simulink model "codd_pfb_fir_4096ch_core"  (R2013b)
settings: Solver=ode45  StartTime=0.0  StopTime=10.0  RelTol=1e-3
undefined symbols (not defined in the file): pfb_coeff_gen_calc
libraries: xbsIndex_r4 x1491, casper_library_misc x112
(part 1 of 18)
settings Model: Creator=ptcs  LastModifiedBy=peix
settings OptimizationCC: ExpressionDepthLimit=2147483647
settings DebuggingCC: StateNameClashWarn=warning

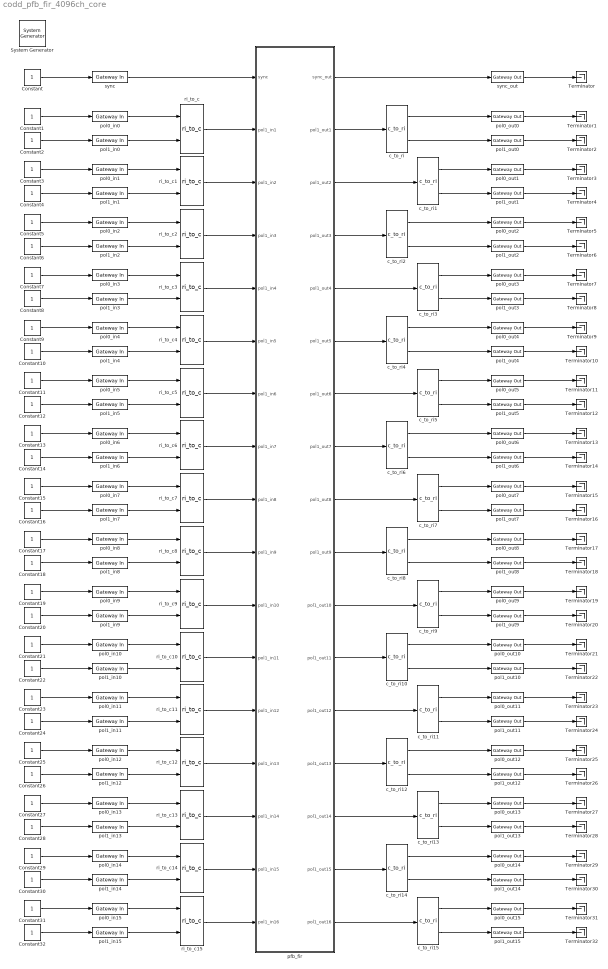
== system codd_pfb_fir_4096ch_core ==
  " System Generator" : xbsIndex_r4/ System Generator  Tag=genX  xilinxfamily=virtex6  part=xc6vsx475t  speed=-1  package=ff1759  synthesis_tool=XST  clock_wrapper=Clock Enables  directory=./codd_pfb_fir_4096ch_core  proj_type=Project Navigator  Synth_file=XST Defaults  Impl_file=ISE Defaults  testbench=off  simulink_period=1  sysclk_period=5.3333  dcm_input_clock_period=100  incr_netlist=off  trim_vbits=Everywhere in SubSystem  dbl_ovrd=According to Block Masks  core_generation=According to Block Masks  run_coregen=off  deprecated_control=off  eval_field=0  block_type=sysgen
  Constant{,1..32} (33 alike) : Constant
  Terminator{,1..32} (33 alike) : Terminator
  c_to_ri{,1..15} (16 alike) : casper_library_misc/c_to_ri  n_bits=18  bin_pt=17
  pfb_fir : Subsystem  Tag=casper:pfb_fir  AncestorBlock=casper_library_pfbs/pfb_fir  mask(pfb_fir){PFBSize=13, TotalTaps=4, WindowType=hamming, n_inputs=4, MakeBiplex=off, BitWidthIn=8, BitWidthOut=18, CoeffBitWidth=18, CoeffDistMem=off, add_latency=1, mult_latency=2, bram_latency=3, fan_latency=2, quantization=Round  (unbiased: Even Values), fwidth=1, mult_spec=2, coeffs_share=on}
      mask prompts: PFBSize "Size of PFB: (2^? pnts)"; TotalTaps "Total Number of Taps:"; WindowType "Windowing Function:"; n_inputs "Number of Simultaneous Inputs: (2^?)"; MakeBiplex "Make Biplex?"; BitWidthIn "Input Bitwidth:"; BitWidthOut "Output Bitwidth:"; CoeffBitWidth "Coefficient Bitwidth:"; CoeffDistMem "Use Distributed Memory for Coeffs"; add_latency "Add Latency"; mult_latency "Mult Latency"; bram_latency "BRAM Latency"; fan_latency "Fanout Latency"; quantization "Quantization Behavior"; fwidth "Bin Width Scaling (normal=1)"; mult_spec "Multiplier specification (0=core, 1=embedded, 2=behavioural) (left=1st tap, or just one value)"; coeffs_share "Share coefficients between polarisations (use less BRAM)?"
      mask init:
      | pfb_fir_init(gcb, ...
      |     'PFBSize', PFBSize, ...
      |     'TotalTaps', TotalTaps, ...
      |     'WindowType', WindowType, ...
      |     'n_inputs', n_inputs, ...
      |     'MakeBiplex', MakeBiplex, ...
      |     'BitWidthIn', BitWidthIn, ...
      |     'BitWidthOut', BitWidthOut, ...
      |     'CoeffBitWidth', CoeffBitWidth, ...
      |     'CoeffDistMem', CoeffDistMem, ...
      |     'add_latency', add_latency, ...
      |     'mult_latency', mult_latency, ...
      |     'bram_latency', bram_latency, ...
      |     'fan_latency', fan_latency, ...
      |     'quantization', quantization, ...
      |     'fwidth', fwidth, ...
      |     'mult_spec', mult_spec, ...
      |     'coeffs_share', coeffs_share);
      settings: AttributesFormatString=|
      | taps=4, add_latency=1
      | max scale 0.596
      mask Help: eval('xlWeb(''http://casper.berkeley.edu/wiki/Pfb_fir'')')
      mask Callback TotalTaps:
      | %num_taps = eval(get_param(gcb, 'TotalTaps'));
      | %old_vec = eval(get_param(gcb, 'mult_spec'));
      | 
      | %vec = 2.*ones(1,num_taps);
      | %old_size = length(old_vec);
      | 
      | %if(old_size <= num_taps),
      | %   new_size = old_size;
      | %else,
      | %    new_size = num_taps;
      | %end
      | 
      | %for n = 1:new_size, vec(n) = old_vec(n); end
      | %set_param(gcb, 'mult_spec', mat2str(vec));
      mask TypeOptions WindowType: bartlett | barthannwin | blackman | blackmanharris | bohamwin | chebwin | flattopwin | gausswin | hamming | hann | kaiser | nuttallwin | parzenwin | rectwin | tukeywin | triang | userwindow
      mask TypeOptions quantization: Truncate | Round  (unbiased: +/- Inf) | Round  (unbiased: Even Values)
      mask Callback fwidth:
      | %num_taps = eval(get_param(gcb, 'TotalTaps'));
      | %old_vec = eval(get_param(gcb, 'mult_spec'));
      | 
      | %vec = 2.*ones(1,num_taps);
      | %old_size = length(old_vec);
      | 
      | %if(old_size <= num_taps),
      | %    new_size = old_size;
      | %else,
      | %    new_size = num_taps;
      | %end
      | 
      | %for n = 1:new_size, vec(n) = old_vec(n); end
      | %set_param(gcb, 'mult_spec', mat2str(vec));
      mask Callback mult_spec:
      | %num_taps = eval(get_param(gcb, 'TotalTaps'));
      | %old_vec = eval(get_param(gcb, 'mult_spec'));
      | 
      | %vec = 2.*ones(1,num_taps);
      | %old_size = length(old_vec);
      | 
      | %if(old_size <= num_taps),
      | %    new_size = old_size;
      | %else,
      | %    new_size = num_taps;
      | %end
      | 
      | %for n = 1:new_size, vec(n) = old_vec(n); end
      | %set_param(gcb, 'mult_spec', mat2str(vec));
  pol0_in{0..15} (16 alike) : xbsIndex_r4/Gateway In  gui_display_data_type=Fixed-point  arith_type="Signed  (2's comp)"  n_bits=8  bin_pt=7  preci_type=Single  exp_width=8  frac_width=24  quantization="Round  (unbiased: +/- Inf)"  overflow=Saturate  period=1  dbl_ovrd=off  timing_constraint=None  locs_specified=off  LOCs={}  UseAsADC=off  ADCChannel='1'  inherit_from_input=off  hdl_port=on  block_type=gatewayin
  pol0_out{0..15} (16 alike) : xbsIndex_r4/Gateway Out  inherit_from_input=off  hdl_port=on  timing_constraint=None  locs_specified=off  LOCs={}  UseAsDAC=off  DACChannel='1'  block_type=gatewayout
  pol1_in{0..15} (16 alike) : xbsIndex_r4/Gateway In  gui_display_data_type=Fixed-point  arith_type="Signed  (2's comp)"  n_bits=8  bin_pt=7  preci_type=Single  exp_width=8  frac_width=24  quantization="Round  (unbiased: +/- Inf)"  overflow=Saturate  period=1  dbl_ovrd=off  timing_constraint=None  locs_specified=off  LOCs={}  UseAsADC=off  ADCChannel='1'  inherit_from_input=off  hdl_port=on  block_type=gatewayin
  pol1_out{0..15} (16 alike) : xbsIndex_r4/Gateway Out  inherit_from_input=off  hdl_port=on  timing_constraint=None  locs_specified=off  LOCs={}  UseAsDAC=off  DACChannel='1'  block_type=gatewayout
  ri_to_c{,1..15} (16 alike) : casper_library_misc/ri_to_c
  sync : xbsIndex_r4/Gateway In  gui_display_data_type=Boolean  arith_type=Boolean  n_bits=16  bin_pt=14  preci_type=Single  exp_width=8  frac_width=24  quantization="Round  (unbiased: +/- Inf)"  overflow=Saturate  period=1  dbl_ovrd=off  timing_constraint=None  locs_specified=off  LOCs={}  UseAsADC=off  ADCChannel='1'  inherit_from_input=off  hdl_port=on  block_type=gatewayin
  sync_out : xbsIndex_r4/Gateway Out  inherit_from_input=off  hdl_port=on  timing_constraint=None  locs_specified=off  LOCs={}  UseAsDAC=off  DACChannel='1'  block_type=gatewayout
  wires:
  pol0_in0/1 -> ri_to_c/1
  pol1_in0/1 -> ri_to_c/2
  ri_to_c/1 -> pfb_fir/2(pol1_in1)
  sync/1 -> pfb_fir/1(sync)
  ri_to_c2/1 -> pfb_fir/4(pol1_in3)
  pol0_in1/1 -> ri_to_c1/1
  pol1_in1/1 -> ri_to_c1/2
  pol0_in2/1 -> ri_to_c2/1
  pol1_in2/1 -> ri_to_c2/2
  ri_to_c1/1 -> pfb_fir/3(pol1_in2)
  ri_to_c3/1 -> pfb_fir/5(pol1_in4)
  pol0_in3/1 -> ri_to_c3/1
  pol1_in3/1 -> ri_to_c3/2
  ri_to_c4/1 -> pfb_fir/6(pol1_in5)
  pol0_in4/1 -> ri_to_c4/1
  pol1_in4/1 -> ri_to_c4/2
  ri_to_c5/1 -> pfb_fir/7(pol1_in6)
  pol0_in5/1 -> ri_to_c5/1
  pol1_in5/1 -> ri_to_c5/2
  ri_to_c6/1 -> pfb_fir/8(pol1_in7)
  pol0_in6/1 -> ri_to_c6/1
  pol1_in6/1 -> ri_to_c6/2
  ri_to_c7/1 -> pfb_fir/9(pol1_in8)
  pol0_in7/1 -> ri_to_c7/1
  pol1_in7/1 -> ri_to_c7/2
  ri_to_c8/1 -> pfb_fir/10(pol1_in9)
  pol0_in8/1 -> ri_to_c8/1
  pol1_in8/1 -> ri_to_c8/2
  ri_to_c9/1 -> pfb_fir/11(pol1_in10)
  pol0_in9/1 -> ri_to_c9/1
  pol1_in9/1 -> ri_to_c9/2
  ri_to_c10/1 -> pfb_fir/12(pol1_in11)
  pol0_in10/1 -> ri_to_c10/1
  pol1_in10/1 -> ri_to_c10/2
  ri_to_c11/1 -> pfb_fir/13(pol1_in12)
  pol0_in11/1 -> ri_to_c11/1
  pol1_in11/1 -> ri_to_c11/2
  ri_to_c12/1 -> pfb_fir/14(pol1_in13)
  pol0_in12/1 -> ri_to_c12/1
  pol1_in12/1 -> ri_to_c12/2
  ri_to_c13/1 -> pfb_fir/15(pol1_in14)
  pol0_in13/1 -> ri_to_c13/1
  pol1_in13/1 -> ri_to_c13/2
  ri_to_c14/1 -> pfb_fir/16(pol1_in15)
  pol0_in14/1 -> ri_to_c14/1
  pol1_in14/1 -> ri_to_c14/2
  ri_to_c15/1 -> pfb_fir/17(pol1_in16)
  pol0_in15/1 -> ri_to_c15/1
  pol1_in15/1 -> ri_to_c15/2
  pfb_fir/2(pol1_out1) -> c_to_ri/1
  pfb_fir/3(pol1_out2) -> c_to_ri1/1
  pfb_fir/4(pol1_out3) -> c_to_ri2/1
  pfb_fir/5(pol1_out4) -> c_to_ri3/1
  pfb_fir/6(pol1_out5) -> c_to_ri4/1
  pfb_fir/7(pol1_out6) -> c_to_ri5/1
  pfb_fir/8(pol1_out7) -> c_to_ri6/1
  pfb_fir/9(pol1_out8) -> c_to_ri7/1
  pfb_fir/10(pol1_out9) -> c_to_ri8/1
  pfb_fir/11(pol1_out10) -> c_to_ri9/1
  pfb_fir/12(pol1_out11) -> c_to_ri10/1
  pfb_fir/13(pol1_out12) -> c_to_ri11/1
  pfb_fir/14(pol1_out13) -> c_to_ri12/1
  pfb_fir/15(pol1_out14) -> c_to_ri13/1
  pfb_fir/16(pol1_out15) -> c_to_ri14/1
  pfb_fir/17(pol1_out16) -> c_to_ri15/1
  c_to_ri/1 -> pol0_out0/1
  c_to_ri/2 -> pol1_out0/1
  pfb_fir/1(sync_out) -> sync_out/1
  c_to_ri1/1 -> pol0_out1/1
  c_to_ri2/1 -> pol0_out2/1
  c_to_ri3/1 -> pol0_out3/1
  c_to_ri4/1 -> pol0_out4/1
  c_to_ri5/1 -> pol0_out5/1
  c_to_ri6/1 -> pol0_out6/1
  c_to_ri7/1 -> pol0_out7/1
  c_to_ri8/1 -> pol0_out8/1
  c_to_ri9/1 -> pol0_out9/1
  c_to_ri10/1 -> pol0_out10/1
  c_to_ri11/1 -> pol0_out11/1
  c_to_ri1/2 -> pol1_out1/1
  c_to_ri2/2 -> pol1_out2/1
  c_to_ri3/2 -> pol1_out3/1
  c_to_ri4/2 -> pol1_out4/1
  c_to_ri5/2 -> pol1_out5/1
  c_to_ri6/2 -> pol1_out6/1
  c_to_ri7/2 -> pol1_out7/1
  c_to_ri8/2 -> pol1_out8/1
  c_to_ri9/2 -> pol1_out9/1
  c_to_ri10/2 -> pol1_out10/1
  c_to_ri11/2 -> pol1_out11/1
  c_to_ri12/1 -> pol0_out12/1
  c_to_ri12/2 -> pol1_out12/1
  c_to_ri13/1 -> pol0_out13/1
  c_to_ri13/2 -> pol1_out13/1
  c_to_ri14/1 -> pol0_out14/1
  c_to_ri14/2 -> pol1_out14/1
  c_to_ri15/1 -> pol0_out15/1
  c_to_ri15/2 -> pol1_out15/1
  Constant/1 -> sync/1
  Constant1/1 -> pol0_in0/1
  Constant2/1 -> pol1_in0/1
  Constant3/1 -> pol0_in1/1
  Constant4/1 -> pol1_in1/1
  Constant5/1 -> pol0_in2/1
  Constant6/1 -> pol1_in2/1
  Constant7/1 -> pol0_in3/1
  Constant8/1 -> pol1_in3/1
  Constant9/1 -> pol0_in4/1
  Constant10/1 -> pol1_in4/1
  Constant11/1 -> pol0_in5/1
  Constant12/1 -> pol1_in5/1
  Constant13/1 -> pol0_in6/1
  Constant14/1 -> pol1_in6/1
  Constant15/1 -> pol0_in7/1
  Constant16/1 -> pol1_in7/1
  Constant17/1 -> pol0_in8/1
  Constant18/1 -> pol1_in8/1
  Constant19/1 -> pol0_in9/1
  Constant20/1 -> pol1_in9/1
  Constant21/1 -> pol0_in10/1
  Constant22/1 -> pol1_in10/1
  Constant23/1 -> pol0_in11/1
  Constant24/1 -> pol1_in11/1
  Constant25/1 -> pol0_in12/1
  Constant26/1 -> pol1_in12/1
  Constant27/1 -> pol0_in13/1
  Constant28/1 -> pol1_in13/1
  Constant29/1 -> pol0_in14/1
  Constant30/1 -> pol1_in14/1
  Constant31/1 -> pol0_in15/1
  Constant32/1 -> pol1_in15/1
  sync_out/1 -> Terminator/1
  pol0_out0/1 -> Terminator1/1
  pol1_out0/1 -> Terminator2/1
  pol0_out1/1 -> Terminator3/1
  pol1_out1/1 -> Terminator4/1
  pol0_out2/1 -> Terminator5/1
  pol1_out2/1 -> Terminator6/1
  pol0_out3/1 -> Terminator7/1
  pol1_out3/1 -> Terminator8/1
  pol0_out4/1 -> Terminator9/1
  pol1_out4/1 -> Terminator10/1
  pol0_out5/1 -> Terminator11/1
  pol1_out5/1 -> Terminator12/1
  pol0_out6/1 -> Terminator13/1
  pol1_out6/1 -> Terminator14/1
  pol0_out7/1 -> Terminator15/1
  pol1_out7/1 -> Terminator16/1
  pol0_out8/1 -> Terminator17/1
  pol1_out8/1 -> Terminator18/1
  pol0_out9/1 -> Terminator19/1
  pol1_out9/1 -> Terminator20/1
  pol0_out10/1 -> Terminator21/1
  pol1_out10/1 -> Terminator22/1
  pol0_out11/1 -> Terminator23/1
  pol1_out11/1 -> Terminator24/1
  pol0_out12/1 -> Terminator25/1
  pol1_out12/1 -> Terminator26/1
  pol0_out13/1 -> Terminator27/1
  pol1_out13/1 -> Terminator28/1
  pol0_out14/1 -> Terminator29/1
  pol1_out14/1 -> Terminator30/1
  pol0_out15/1 -> Terminator31/1
  pol1_out15/1 -> Terminator32/1
